simulink model "alpha_beta"  (Simulink 7.6)
settings: Solver=FixedStepDiscrete  StartTime=0.0  StopTime=10.0  FixedStep=dt  RelTol=1e-3
undefined symbols (not defined in the file): alpha, beta, dt
settings Model: Creator=sawmilkd  LastModifiedBy=sawmilkd

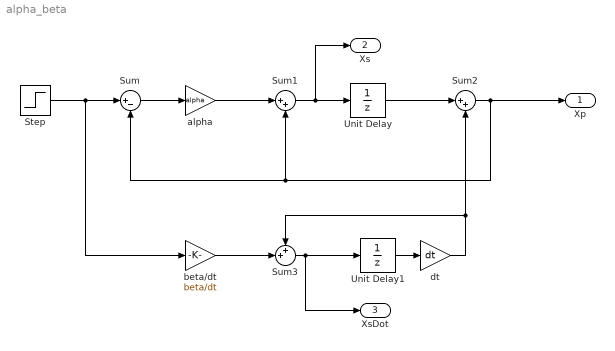
== system alpha_beta ==
  Step : Step  SampleTime=0
  Sum : Sum  Inputs=|+-
  Sum1 : Sum  Inputs=|++
  Sum2 : Sum  Inputs=|++
  Sum3 : Sum  Inputs=++|
  Unit Delay : UnitDelay  SampleTime=-1
  Unit Delay1 : UnitDelay  SampleTime=-1
  alpha : Gain  Gain=alpha
  beta/dt : Gain  Gain=beta/dt
  dt : Gain  Gain=dt
  Xp : Outport
  Xs : Outport  Port=2
  XsDot : Outport  Port=3
  wires:
  Step/1 -> Sum/1, beta/dt/1
  Sum/1 -> alpha/1
  alpha/1 -> Sum1/1
  Sum1/1 -> Unit Delay/1, Xs/1
  Unit Delay/1 -> Sum2/1
  Sum2/1 -> Xp/1, Sum1/2, Sum/2
  beta/dt/1 -> Sum3/2
  Sum3/1 -> Unit Delay1/1, XsDot/1
  Unit Delay1/1 -> dt/1
  dt/1 -> Sum2/2, Sum3/1
